simulink model "Vehicle_Model_Controller_Mar18"  (R2020b)
settings: Solver=VariableStepAuto  StartTime=0.0  StopTime=27  FixedStep=0.015  MaxStep=0.015  RelTol=1e-3
model workspace (MAT data in the model file):
  Kp = 10
  understeer_gradient = 0.05
undefined symbols (not defined in the file): a, A1, A2, b, B1, B2, B3, brakecoeff, c, C1, C2, C3, C4, C_param, d, DiscIntNeverNeededParam, driver_gain, FZ_C, g, gearbox_efficiency, gr, I, inch2mm, J_z, k_limit, Ku, l, max_yaw_field, mech_brake, min_speed_regen, motor_efficiency, motor_limit_power, motor_limit_torque, mu_factor, P, ramp_rate, RE, s, S1, S2, S3, S4, steer_slope, steering_freq, T, T2F, tau, time_delay, V_target
libraries: fl_lib x32, nesl_utility x24, sdl_lib x8, pid_lib x1, autolibshared x1, autolibdatasheetbattery x1
(part 3 of 3)

== matlab function Vehicle_Model_Controller_Mar18/Driver Input Logic/Torque Vectoring Controller/LP_Calc  ==
  settings: updateMethod=DISCRETE
  data: prev_torque input; Tx_actual output double size=[4 1]; driver_input input; FY input; omega_m input; y input; omega_m output; J_z parameter; min_speed_regen parameter; power output double size=[1]; bigM_flag output size=[1]; typed output size=[1]; yaw_accel output double size=[1]; lb input; ub input; A input; b input; Aeq input; beq input; T2F parameter
function [Tx_actual, omega_m, power, bigM_flag, typed, yaw_accel] = LP_calc(prev_torque, driver_input, FY, omega_m, y, J_z, min_speed_regen, lb, ub, A, b, Aeq, beq, T2F)
%% LP_calc Computation
% Developer(s):    David Farell
%                  Demetrius Gulewicz
%                  Elliot Stockwell
%                  Tao Sun
%
% Developed for: Purdue Electric Racing
% Date:          12/25/2021
%
% Description: This function primarily computes the desired torque
%              distribution after constructing an optimization statement.
%
%
%% Pass Through Signals
% omega_m - Motor Shaft Angular Velocity [rad/s][1x4]
%
%
%% Input Only
% prev_torque - Torque Requested To Motor In Previous Time Step [Nm][4x1]
% driver_input - Proportion of total available power to use [Unitless][1x1]
% T2F - Convert Torque At The Motor Shaft to Force At The Tire [1/m][1x4]
% power_limit_battery - Max & Min Total Battery Power Output [W][1x2]
% FY - Tires Forces y Direction, Tire fixed coordinates [N][1x4]
% x - Equivalent Distances That FX Acts From CoG [m][1x4]
% y - Equivalent Distances That FY Acts From CoG [m][1x4]
% slip_limit - Max Torque Before Tire Slips [Nm][1x4]
% torque_limit_motor - Max Torque Motor Can Output [Nm][1x4]
% tau_limit_upper - Max Torque Motor Is Allowed To Change To [Nm][1x4]
% tau_limit_lower - Min Torque Motor Is Allowed To Change To [Nm][1x4]
% PID - Desired Yaw Acceleration [rad/s^2][1x1]
%
%
%% Output Only
% Tx - Torque Request To Motors [Nm][4x1]
% lb - Min Torque Request [Nm][1x4]
% ub - Max Torque Request [Nm][1x4]
% Aeq - Moment About CoG, Optimization Variable [rad/s^2][1x1]
% beq - Moment About CoG, Yaw Acceleration & Other Foces [rad/s^2][1x1]
% A - Power Consumed, Optimization Variable [W][1x1]
% b - Power Consumed, Driver Input [W][1x1]
% M_max - Max & Min Yaw Acceleration Achievable With lb & ub [rad/s^2][1x2]
% Power - Total Estimated Power Consumed by the 4 Motors
% TR - The Estimated Yaw Acceleration from the Vehicle
%
%
%% Constants
% global J_z; % Polar Moment Of Inertia [kg m^2][1x1]
% global motor_efficiency; % Motor efficiency [Unitless][1x4]
% global motor_limit_torque; % Minimum & Max Torque Request From Motor [Nm][1x2]
% global min_speed_regen; % Min Motor Shaft Speed For Regen Braking [rad/s][1x1]
% T2F - Convert Torque At The Motor Shaft to Force At The Tire [1/m][1x4]


%% Detect Potential Zero Crossing, Determine Augmented lb and ub
lb_plus = lb;
ub_neg = ub;
zero_crossing = 0;
crossing_locations = [0 0 0 0];
yaw_error_limit = 0.2;

for i = 1:4
    if lb_plus(i) < 0 && ub_neg(i) > 0
        zero_crossing = 1;
        crossing_locations(i) = i;
        
        if sign(prev_torque(i)) > 0
            lb_plus(i) = 0.001;
        elseif sign(prev_torque(i)) < 0
            ub_neg(i) = -0.001;          
        end
    elseif abs(ub(i) - lb(i)) < 0.5
        ub_neg(i) = -0.001; 
        lb_plus(i) = -10;
        lb(i) = -0.002;
        ub(i) = 0.002;
    end
end

signs = sign(lb_plus);
             
%% Optimization
Tx = single([0 0 0 0]);
bigM_flag = single(0);
typed = 0;
ub_adjust = [0 0 0 0];
lb_adjust = [0 0 0 0];

signs_adjust = [0 0 0 0];

if driver_input < 0
    T2F_aug = -T2F;
    A = -A;
else
    T2F_aug = T2F;
end

if ~(omega_m(1) < min_speed_regen && driver_input < 0)
    if (zero_crossing == 1 && omega_m(1) > 10)
            % Zero Crossing Primary Optimization
            [Tx21, Tx22, Tx23, Tx24, bigM_flag2] = call_bigM_C(T2F_aug, b, A, beq, Aeq, lb_plus, ub_neg, signs, yaw_error_limit);           
            Tx2 = double([Tx21, Tx22, Tx23, Tx24]);
            
            for i = 1:4
                if abs(Tx2(i)) < 0.002 && abs(Tx2(i)) >= 0.001 && crossing_locations(i) > 0
                    if signs(i) > 0
                        lb_adjust(i) = lb(i);
                        ub_adjust(i) = -lb_plus(i);
                    else
                        lb_adjust(i) = -ub_neg(i);
                        ub_adjust(i) = ub(i);  
                    end
                elseif crossing_locations(i) > 0
                    lb_adjust(i) = lb_plus(i);
                    ub_adjust(i) = ub_neg(i);
                else
                    lb_adjust(i) = lb(i);
                    ub_adjust(i) = ub(i);
                end
            end
            
            signs_adjust = sign(lb_adjust);
            [Tx31, Tx32, Tx33, Tx34, bigM_flag3] = call_bigM_C(T2F_aug, b, A, beq, Aeq, lb_adjust, ub_adjust, signs_adjust, yaw_error_limit);
            Tx3 = double([Tx31, Tx32, Tx33, Tx34]);
            
            % Zero Crossing Secondary Optimization
            [Tx5, bigM_flag5] = call_bigM_alt(b, A, beq, Aeq, lb, ub_neg);
            
            for i = 1:4
                if abs(Tx5(i)) < 0.002 && abs(Tx5(i)) >= 0.001 && crossing_locations(i) > 0
                    if signs(i) > 0
                        lb_adjust(i) = lb(i);
                        ub_adjust(i) = -lb_plus(i);
                    else
                        lb_adjust(i) = -ub_neg(i);
                        ub_adjust(i) = ub(i);  
                    end
                elseif crossing_locations(i) > 0
                    lb_adjust(i) = lb_plus(i);
                    ub_adjust(i) = ub_neg(i);
                else
                    lb_adjust(i) = lb(i);
                    ub_adjust(i) = ub(i);
                end
            end
            
            [Tx6, bigM_flag6] = call_bigM_alt(b, A, beq, Aeq, lb_adjust, ub_adjust);
            
            % Optimization Selection
            if bigM_flag3 == 1 || bigM_flag3 == 3
                Tx = single(Tx3);
                typed = 3;
                bigM_flag = single(bigM_flag3);
            else
                Tx = single(Tx6);
                typed = 6;
                bigM_flag = single(bigM_flag6);
            end
    else    
        % No Zero Crossing
        [Tx11, Tx12, Tx13, Tx14, bigM_flag1] = call_bigM_C(T2F_aug, b, A, beq, Aeq, lb, ub, signs, 0.05);
        Tx1 = [Tx11, Tx12, Tx13, Tx14];
        [Tx4, bigM_flag4] = call_bigM_alt(b, A, beq, Aeq, lb, ub);
        
        % Optimization Selection
        if bigM_flag1 == 3 || bigM_flag1 == 1
            Tx = single(Tx1);
            typed = 1;
            bigM_flag = single(bigM_flag1);
        else
            Tx = single(Tx4);
            typed = 4;
            bigM_flag = single(bigM_flag4);
        end   
    end
else
    typed = 7;
    bigM_flag = single(3);
end

Tx_actual = double(Tx');
yaw_accel = double((sum(Aeq.*Tx_actual')+sum(y.*FY/J_z)));
power = double(sum(Tx_actual' .* sign(driver_input).*A));


%% Simplified Control Scheme
% Tx_actual = driver_input .* [25; 25; 25; 25];


end

== matlab function Vehicle_Model_Controller_Mar18/Motor and Battery/Motors/   ==
  data: Battery_Voltage input; ang_vel_RAD input; battery_current output; Motor_torque input; battery_power output
function [battery_current, battery_power]= get_batt_curr(Battery_Voltage, ang_vel_RAD, Motor_torque)
%% Current Draw
% Developers:    Demetrius Gulewicz

% Developed for: Purdue Electric Racing
% Date:          09/18/2021
%
% Definitions:
% ang_vel_RAD:   Angular velocity of each wheel on the wheel fixed y axis [RAD]
% Motor_torque:  Torque the motor actually outputs                 [Ncm]
% Battery_Voltage: The voltage of the battery                      [V]

%% Definitions
a = 0.0411;
b = 2.7976;
c = 45.978;

t = Motor_torque;
w = ang_vel_RAD;
v = Battery_Voltage;

e = 85;

%% Calculate Current Draw
%x0 = [20, 20, 20, 20];
%options = optimoptions('fsolve','Algorithm','Levenberg-Marquardt');
%F = @(x) ([(a * x(1)^3) + (b * x(1)^2) + (c * x(1)), ] .* v) - (t .* w);
%battery_current = sum(fsolve(F,x0,options));

battery_current = sum((t .* w) ./ (e .* v));
battery_power = battery_current * Battery_Voltage;
end
